simulink model "GEMV_Ex5"  (R2025a)
settings: Solver=VariableStepAuto  StartTime=0.0  StopTime=100  RelTol=1e-3
undefined symbols (not defined in the file): Column, DUT, GEMV_Ex1_Stream, L, major, vsva1596, xcvc1702
libraries: aieUtilities x2, aieDSP x1, vmcUtilities x1
settings Model: Creator=sdegala  LastModifiedBy=robg
settings ModelReferenceCC: EnableRefExpFcnMdlSchedulingChecks=on
settings RTWCC: GPUComputeCapability=3.5

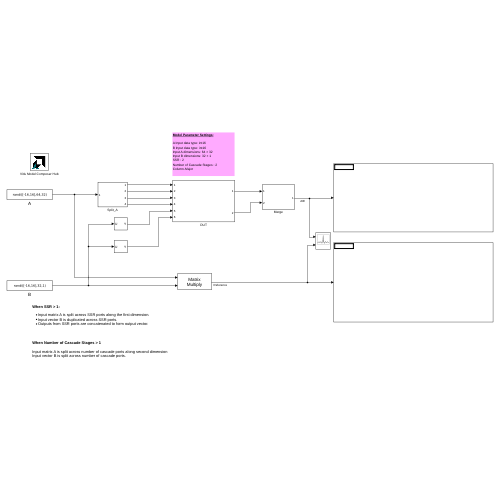
[thumbnail: Simulink's stored preview of the top-level diagram]
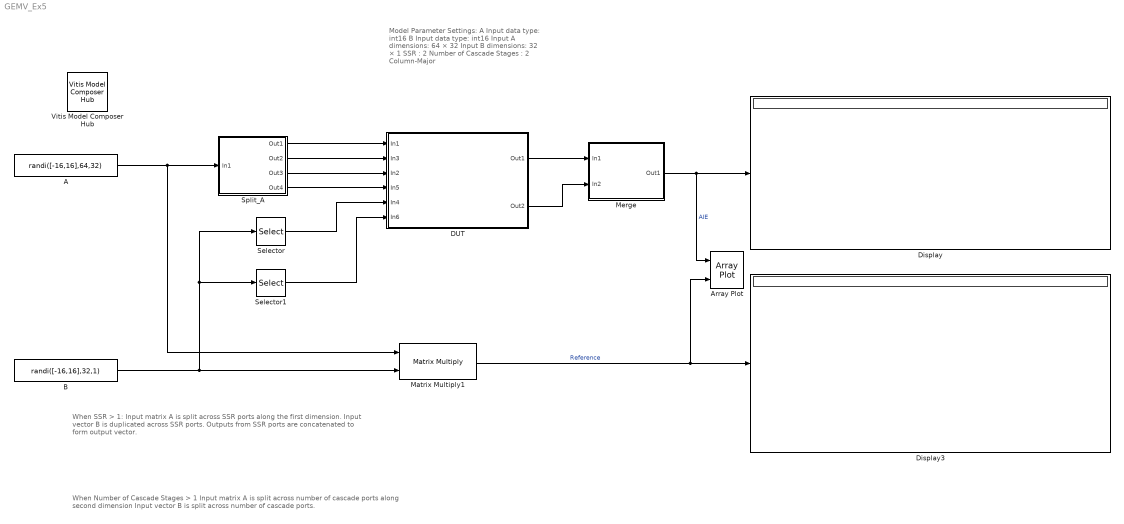
== system GEMV_Ex5 ==
  note: When Number of Cascade Stages > 1
      |
      | Input matrix A is split across number of cascade ports along second dimension
      | Input vector B is split across number of cascade ports.
  note: When SSR > 1:
      | Input matrix A is split across SSR ports along the first dimension.
      | Input vector B is duplicated across SSR ports.
      | Outputs from SSR ports are concatenated to form output vector.
  note: Model Parameter Settings:
      |
      | A Input data type: int16
      | B Input data type: int16
      | Input A dimensions: 64 × 32
      | Input B dimensions: 32 × 1
      | SSR : 2
      | Number of Cascade Stages : 2
      | Column-Major
  A : Constant  Value=randi([-16,16],64,32)  OutDataTypeStr=int16  SampleTime=1
  Array Plot : ArrayPlot  NumInputPorts=2  WindowPosition=[734.000000,269.000000,800.000000,500.000000,]  Visible=on  ScopeFrameLocation=window  YLimits=[0.75 13.25]  ShowLegend=on
  B : Constant  Value=randi([-16,16],32,1)  OutDataTypeStr=int16  SampleTime=1
  DUT : Subsystem
  Display : Display
  Display3 : Display
  Matrix Multiply1 : Product  Multiplication=Matrix(*)  OutDataTypeStr=int16
  Merge : Subsystem
  Selector : Selector  InputPortWidth=32  IndexOptions=Index vector (dialog)  Indices=1:2:32  OutputSizes=1
  Selector1 : Selector  InputPortWidth=32  IndexOptions=Index vector (dialog)  Indices=2:2:32  OutputSizes=1
  Split_A : Subsystem
  Vitis Model Composer Hub : vmcUtilities/Vitis Model Composer Hub  Tag=genX  CodeGeneration=off  SubsystemName=DUT  BlockHierPath=GEMV_Ex1_Stream/DUT  SubsystemType=AIENode  StartColumn=1  NumberOfColumns=1  TargetDirectory=./code  exportDesign=off  analyzeDesign=on  validateDesignOnHw=off  ExportType=AI Engines  IpVendor=xilinx.com  IpLibrary=hls  IpVersion=1.0  IpHWLanguage=Verilog  AieCompilerOptions={}  AieSimulatorOptions={}  CreateTestbench=on  TestbenchStackSize=10  RunRtlSim=off  RunCSim=off  RunAieSim=off  enableSimulationTimeout=on  enableGraphIterations=on  AieSimTimeout=50000  AieGraphIterations=-1  RunAieSimProfiling=off  LaunchVitisAnalyzer=off  PlotOutput=off  RunX86Sim=off  X86SimTimeout=10  GenHwImage=off  GenLibadfXo=off  GenHwValidationCode=off  PlatformType=Not Specified  HwSystemType=Baremetal  HwValidationTarget=hw  ProjDevice=xcvc1702-vsva1596-2LP-e-L  ProjDevicePart=xcvc1702-vsva1596-2LP-e-L  AIEType=AIE  SamplePeriod=-1  ClockFrequency=200  DataPathParallelism=1  xilinxfamily=versalaicore  part=xcvc1702  speed=-2LP-e-L  package=vsva1596  directory=./netlist  testbench=off  incr_netlist=off  synthesis_tool=Vivado  clock_wrapper=Clock Enables  dbl_ovrd=According to Block Masks  dcm_input_clock_period=10  sysclk_period=10  simulink_period=1  eval_field=0  IPInfoJsonString="{\"DUTSubsystemName\":\"DUT\",\"AIESubsystem\":{\"SubsystemName\":\"DUT\",\"TargetDirectory\":\"./code\",\"AIEArrayConfig\":\"Use entire AIE array\",\"StartColumn\":\"0\",\"NumberOfColumns\":\"1\"},\"SubsystemTag\":\"AIENode\"}"  LogFileName=/proj/xhdhdstaff5/sdegala/Head1/HEAD/2026_1_Work/code/model_composer.log  NThreads=4  IPConfigFile=/tmp/vmctmp-16505700046410390857/GEMV_Ex1_Stream_ipconfig.json
  wires:
  Split_A/1(Out1) -> DUT/1(In1)
  DUT/1(Out1) -> Merge/1(In1)
  DUT/2(Out2) -> Merge/2(In2)
  Merge/1(Out1) -> Array Plot/1, Display/1  "AIE"
  Matrix Multiply1/1 -> Array Plot/2, Display3/1  "Reference"
  A/1 -> Matrix Multiply1/1, Split_A/1(In1)
  Split_A/3(Out3) -> DUT/3(In2)
  Split_A/4(Out4) -> DUT/4(In5)
  Split_A/2(Out2) -> DUT/2(In3)
  Selector/1 -> DUT/5(In4)
  B/1 -> Matrix Multiply1/2, Selector1/1, Selector/1
  Selector1/1 -> DUT/6(In6)

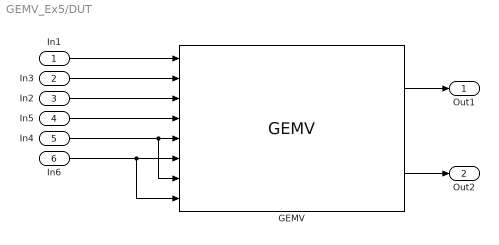
== system GEMV_Ex5/DUT ==
  In1 : Inport
  In3 : Inport  Port=2
  In2 : Inport  Port=3
  In5 : Inport  Port=4
  In4 : Inport  Port=5
  In6 : Inport  Port=6
  GEMV : aieDSP/GEMV  AIE_VARIANT=1  data_type_A=int16  data_type_B=int16  Matrix_reload=off  api=0  Dim_A=64  Dim_B=32  num_frames=1  ssr=2  casc_length=2  dual_ip=off  num_outputs=off  A_Leading_data=Column-major(1)  shift_output=0  rnd_mode=Floor  sat_mode=None  blockJsonConstraints=[]  blockJsonConstraintsInternal=[]  spec=vmc_matrix_vector_mul.json  SerializedMaskParamNames=[]  SerializedMaskParamValues=[]  SerializedMaskParamVisibilities=[]  block_type=GEMV  SerializedMaskParamDataypes=uint|typename|typename|uint|uint|uint|uint|uint|uint|uint|uint|uint|uint|uint|uint|uint  SerializedMaskParamEnumStrArr=0|0|0|0|0|0|0|0|0|0|0|0|Row-major(0),Column-major(1)|0|Floor,Ceiling,Round to positive infinity,Round to negative infinity,Round symmetrical to infinity,Round symmetrical to zero,Round convergent to even,Round convergent to odd|None,Saturate,Symmetric  SerializedMaskParamEnumValArr=0|0|0|0|0|0|0|0|0|0|0|0|0,1|0|0,1,2,3,4,5,6,7|0,1,3  SerializedMaskParamVectorArr=0|0|0|0|0|0|0|0|0|0|0|0|0|0|0|0  SerializedMaskParamKeys=AIE_VARIANT|TT_DATA_A|TT_DATA_B|TP_USE_MATRIX_RELOAD|TP_API|TP_DIM_A|TP_DIM_B|TP_NUM_FRAMES|TP_SSR|TP_CASC_LEN|TP_DUAL_IP|TP_NUM_OUTPUTS|TP_DIM_A_LEADING|TP_SHIFT|TP_RND|TP_SAT
  Out1 : Outport
  Out2 : Outport  Port=2
  wires:
  GEMV/1 -> Out1/1
  GEMV/2 -> Out2/1
  In1/1 -> GEMV/1
  In3/1 -> GEMV/2
  In2/1 -> GEMV/3
  In5/1 -> GEMV/4
  In6/1 -> GEMV/8, GEMV/6
  In4/1 -> GEMV/7, GEMV/5

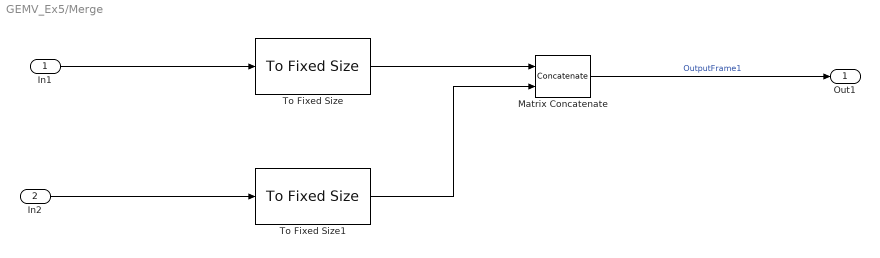
== system GEMV_Ex5/Merge ==
  In1 : Inport
  In2 : Inport  Port=2
  Matrix Concatenate : Concatenate  ConcatenateDimension=2
  To Fixed Size : aieUtilities/To Fixed Size  Mode=Stop simulation when input variable-size signal is not full  OutputSize=Inherit: Same as input  CopyMethod=Buffer samples to form output  HasStatusOutput=on
  To Fixed Size1 : aieUtilities/To Fixed Size  Mode=Stop simulation when input variable-size signal is not full  OutputSize=Inherit: Same as input  CopyMethod=Buffer samples to form output  HasStatusOutput=on
  Out1 : Outport
  wires:
  To Fixed Size/1 -> Matrix Concatenate/1
  To Fixed Size1/1 -> Matrix Concatenate/2
  Matrix Concatenate/1 -> Out1/1  "OutputFrame1"
  In1/1 -> To Fixed Size/1
  In2/1 -> To Fixed Size1/1

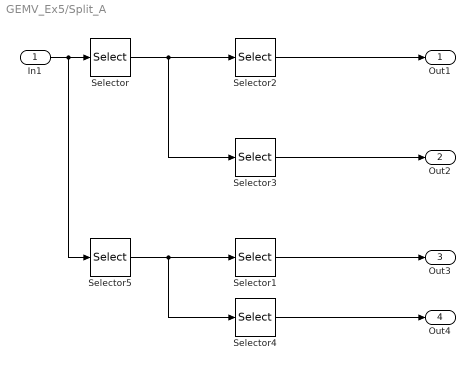
== system GEMV_Ex5/Split_A ==
  In1 : Inport
  Selector : Selector  NumberOfDimensions=2  InputPortWidth=64  IndexOptions=Index vector (dialog),Index vector (dialog)  Indices=1:32,1:1:32  OutputSizes=1,1
  Selector1 : Selector  NumberOfDimensions=2  InputPortWidth=64  IndexOptions=Index vector (dialog),Index vector (dialog)  Indices=1:32,1:2:32  OutputSizes=1,1
  Selector2 : Selector  NumberOfDimensions=2  InputPortWidth=64  IndexOptions=Index vector (dialog),Index vector (dialog)  Indices=1:32,1:2:32  OutputSizes=1,1
  Selector3 : Selector  NumberOfDimensions=2  InputPortWidth=64  IndexOptions=Index vector (dialog),Index vector (dialog)  Indices=1:32,2:2:32  OutputSizes=1,1
  Selector4 : Selector  NumberOfDimensions=2  InputPortWidth=64  IndexOptions=Index vector (dialog),Index vector (dialog)  Indices=1:32,2:2:32  OutputSizes=1,1
  Selector5 : Selector  NumberOfDimensions=2  InputPortWidth=64  IndexOptions=Index vector (dialog),Index vector (dialog)  Indices=33:1:64,1:1:32  OutputSizes=1,1
  Out1 : Outport
  Out2 : Outport  Port=2
  Out3 : Outport  Port=3
  Out4 : Outport  Port=4
  wires:
  Selector2/1 -> Out1/1
  Selector3/1 -> Out2/1
  Selector5/1 -> Selector4/1, Selector1/1
  Selector4/1 -> Out4/1
  Selector1/1 -> Out3/1
  Selector/1 -> Selector3/1, Selector2/1
  In1/1 -> Selector5/1, Selector/1
